simulink model "mconversion7"  (Simulink 8.0)
settings: Solver=FixedStepDiscrete  StartTime=0.0  StopTime=10.0  RelTol=1e-3
settings Model: Creator=awarlock  LastModifiedBy=htu  ExtModeAutoUpdateStatusClock=off
settings DataIOCC: SignalLoggingSaveFormat=ModelDataLogs
settings OptimizationCC: InitFltsAndDblsToZero=on
settings DebuggingCC: SaveWithParameterizedLinksMsg=none  CheckExecutionContextPreStartOutputMsg=on  CheckExecutionContextRuntimeOutputMsg=on  SignalResolutionControl=TryResolveAllWithWarning  MultiTaskDSMMsg=warning  MultiTaskCondExecSysMsg=none
settings RTWCC: IncludeERTFirstTime=on
settings GRTTargetCC: TargetFcnLib=ansi_tfl_tmw.mat  CombineOutputUpdateFcns=off  GRTInterface=on

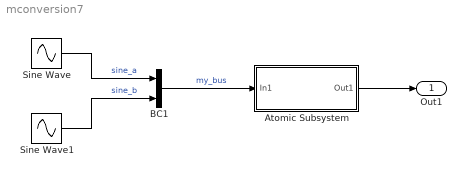
== system mconversion7 ==
  Atomic Subsystem : Subsystem  TreatAsAtomicUnit=on
  BC1 : BusCreator  DialogController=Simulink.DDGSource_Bus  Inputs=2
  Sine Wave : Sin  SineType=Sample based  SampleTime=0.1
  Sine Wave1 : Sin  SampleTime=0.1
  Out1 : Outport
  wires:
  BC1/1 -> Atomic Subsystem/1(In1)  "my_bus"
  Sine Wave/1 -> BC1/1  "sine_a"
  Sine Wave1/1 -> BC1/2  "sine_b"
  Atomic Subsystem/1(Out1) -> Out1/1

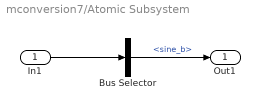
== system mconversion7/Atomic Subsystem ==
  In1 : Inport
  Bus Selector : BusSelector  DialogController=Simulink.DDGSource_Bus  OutputSignals=sine_b
  Out1 : Outport
  wires:
  In1/1 -> Bus Selector/1
  Bus Selector/1 -> Out1/1  "<sine_b>"
